simulink library "opticalComponentLibrary"  (R2014a)
settings: Solver=ode45  StartTime=0.0  StopTime=10.0  RelTol=1e-3
settings Model: Creator=Nithya Menon  LastModifiedBy=Nithya Menon

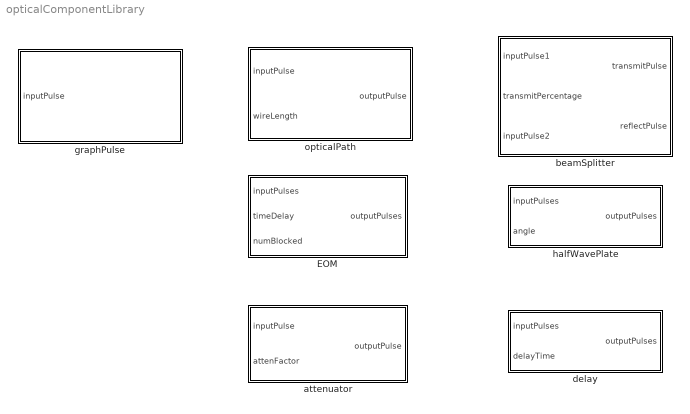
== system opticalComponentLibrary ==
  EOM : MATLAB Function  TreatAsAtomicUnit=on
  attenuator : MATLAB Function  TreatAsAtomicUnit=on
  beamSplitter : MATLAB Function  TreatAsAtomicUnit=on
  delay : MATLAB Function  TreatAsAtomicUnit=on
  graphPulse : MATLAB Function  TreatAsAtomicUnit=on
  halfWavePlate : MATLAB Function  TreatAsAtomicUnit=on
  opticalPath : MATLAB Function  TreatAsAtomicUnit=on

== matlab function opticalComponentLibrary/beamSplitter ==
  data: inputPulse1 input; transmitPulse output; transmitPercentage input; reflectPulse output; inputPulse2 input
function [ transmitPulse, reflectPulse ] = beamSplitter( inputPulse1, transmitPercentage, inputPulse2)
%   Inputs: inputPulse, transmitPercentage (where the percentage reflected
%           is 1 - transmitPercentage) 
%   Outputs: transmitPulse, reflectedPulse measured relative to
%   inputPulses1

transmitPercentage = transmitPercentage/100;

transmitPulse = inputPulse1;
reflectPulse = inputPulse1; 

transmitPulse(:,2) = transmitPulse(:,2)*transmitPercentage;
reflectPulse(:,2) = reflectPulse(:,2)*(1-transmitPercentage);


if size(inputPulse2,1) > 1, 
    transmitPulse2 = inputPulse2;
    reflectPulse2 = inputPulse2; 

    transmitPulse2(:,2) = transmitPulse2(:,2)*transmitPercentage;
    reflectPulse2(:,2) = reflectPulse2(:,2)*(1-transmitPercentage);
    
%     the reflected pulse of the second input follows the path of the
%     transmited first input pulse, and the transmited pulse of the second input
%     follows the path of the reflected first input pulse
    transmitPulse = transmitPulse + reflectPulse2;
    reflectPulse = transmitPulse + transmitPulse2; 
end

end

== matlab function opticalComponentLibrary/opticalPath ==
  data: inputPulse input; outputPulse output; wireLength input
function outputPulse   = opticalPath( inputPulse, wireLength )
%   Inputs: inputPulse [frequency, power, offset, polarization],
%           wireLength (meters)
%   Outputs: modulated output pulse

outputPulse = inputPulse;

wireDelay = (wireLength / (2.99792458 * 10^8));
timeStepsToShift = wireDelay / inputPulse(2,1);
% impulseResponse = [zeros(1, timeStepsToShift) 1];
impulseResponse = [zeros(1,600)  1];
convolved = conv(inputPulse(:,2), impulseResponse);
outputPulse(:,2) = convolved(1:size(inputPulse,1));

end

== matlab function opticalComponentLibrary/EOM ==
  data: inputPulses input; outputPulses output; timeDelay input; numBlocked input
function outputPulses   = EOM( inputPulses, timeDelay, numBlocked)
%   Inputs: inputPulses - A list of input pulses
%           numBlocked - number of blocked pulses 
%   Outputs: outputPulses - delayed output pulses
%

[nrow, ncol] = size(inputPulses);
outputPulses = zeros([nrow,ncol]);

numBlocked = numBlocked+1;

for i = 1:nrow
    currentPulse = inputPulses(i,:);
    currentPulse(1) = currentPulse(1)/numBlocked; % computes delay in ns
    currentPulse(3) = currentPulse(3) + timeDelay;
    outputPulses(i,:) = currentPulse;   
end



%plotPulses = [outputPulses; inputPulses];
%pulseSequenceDisplay(plotPulses, 0.3*10^(-6))

== matlab function opticalComponentLibrary/halfWavePlate ==
  data: inputPulses input; outputPulses output; angle input
function outputPulses   = halfWavePlate( inputPulses, angle)
%   Input: inputPulse, angle (between polarization vector and direction of
%          propagation along the waveplate's fast axis)
%   Output: outputPulse

[nrow, ncol] = size(inputPulses);
outputPulses = [];
for i = 1:nrow,
    currentPulse = inputPulses(i,:);
    if currentPulse(4) == 0 && angle == 45; % vertical polarization
        currentPulse(4) = 1;
    elseif currentPulse(4) == 1 && angle == 45; % horizontal polarization
        currentPulse(4) = 0;
    end
    outputPulses = [outputPulses; currentPulse];
end

== matlab function opticalComponentLibrary/attenuator ==
  data: inputPulse input; outputPulse output; attenFactor input
function outputPulse   = attenuate( inputPulse, attenFactor)
%   Inputs: inputPulse - input pulse matrix
%           attenFactor - a specified factor each pulse will be attenuated
%           by
%   Outputs: outputPulse - attenuated output pulse
%
outputPulse = inputPulse;
outputPulse(:,2) = inputPulse(:,2)*1/attenFactor; 


end

== matlab function opticalComponentLibrary/delay ==
  data: inputPulses input; outputPulses output; delayTime input
function outputPulses   = delay( inputPulses, delayTime)
%   Inputs: inputPulses - A list of input pulses
%           delayTime - a specified time in seconds all input pulses will be 
%           delayed by
%   Outputs: outputPulses - delayed output pulses
%
[nrow, ncol] = size(inputPulses);
outputPulses = zeros([nrow,ncol]);

for i = 1:nrow
    currentPulse = inputPulses(i,:);
    currentPulse(3) = delayTime + currentPulse(3); % computes delay in ns
    outputPulses(i,:) = currentPulse;    
end

== matlab function opticalComponentLibrary/graphPulse ==
  data: inputPulse input
function opticalPath(inputPulse)
%   Inputs: inputPulse [ N x 3] matrix containing time, value, and
%           polarization in each row
%   Outputs: plots  time vs. value 

tVector = inputPulse(:,1);
yVector = inputPulse(:,2);

plot(tVector, yVector);


end
